simulink library "passive_control"  (Simulink 7.1)
values from neighbouring files (symbols this model uses):
  sysdsp = feedback(sysdp,Kc)    [calc_sysdsp.m]
  Ts = 1    [calc_sysdsp.m]
undefined symbols (not defined in the file or in its folder): A, B, b, C, D, gravload, Kv, Kx, M, ms, nc, np, q0, tau_passify
libraries: instrumentlib x8, passive_control x4, simulink x4, roblocks x2, dspsigops x2
(part 2 of 2)

== system passive_control/passify/ipesh_vel_est_2 ==
  u : Inport
  Embedded MATLAB Function : Stateflow chart
  Unit Delay : UnitDelay  X0=x0  SampleTime=-1
  y : Outport
  wires:
  Embedded MATLAB Function/1(y) -> y/1
  u/1 -> Embedded MATLAB Function/1(u)
  Unit Delay/1 -> Embedded MATLAB Function/2(x_k)
  Embedded MATLAB Function/2(x_k_p_1) -> Unit Delay/1

== system passive_control/passify/ipesh_vel_est_3 ==
  u : Inport
  Embedded MATLAB Function : Stateflow chart
  Unit Delay : UnitDelay  X0=x0  SampleTime=-1
  y : Outport
  wires:
  Embedded MATLAB Function/2(x_k_p_1) -> Unit Delay/1
  Unit Delay/1 -> Embedded MATLAB Function/2(x_k)
  u/1 -> Embedded MATLAB Function/1(u)
  Embedded MATLAB Function/1(y) -> y/1

== system passive_control/passify/ipesh_vel_est_4 ==
  u : Inport
  Embedded MATLAB Function : Stateflow chart
  Unit Delay : UnitDelay  X0=x0  SampleTime=-1
  y : Outport
  wires:
  Embedded MATLAB Function/1(y) -> y/1
  u/1 -> Embedded MATLAB Function/1(u)
  Unit Delay/1 -> Embedded MATLAB Function/2(x_k)
  Embedded MATLAB Function/2(x_k_p_1) -> Unit Delay/1

== system passive_control/passive_down_sampler/DT_Integrator ==
  In1 : Inport
  Sum2 : Sum  Inputs=|++  OutDataType=sfix(16)  OutScaling=2^0
  Unit Delay : UnitDelay  Orientation=left  SampleTime=-1
  Out1 : Outport
  wires:
  In1/1 -> Sum2/1
  Unit Delay/1 -> Sum2/2
  Sum2/1 -> Out1/1, Unit Delay/1  "sum_1"

== system passive_control/passive_down_sampler/DT_Integrator1 ==
  In1 : Inport
  Sum2 : Sum  Inputs=|++  OutDataType=sfix(16)  OutScaling=2^0
  Unit Delay : UnitDelay  Orientation=left  SampleTime=-1
  Out1 : Outport
  wires:
  Sum2/1 -> Unit Delay/1, Out1/1  "sum_1"
  Unit Delay/1 -> Sum2/2
  In1/1 -> Sum2/1

== system passive_control/trajectory_gen/ipesh_traj ==
  u : Inport
  Embedded MATLAB Function : Stateflow chart
  Unit Delay : UnitDelay  X0=x0  SampleTime=-1
  y : Outport
  wires:
  Embedded MATLAB Function/1(y) -> y/1
  u/1 -> Embedded MATLAB Function/1(u)
  Unit Delay/1 -> Embedded MATLAB Function/2(x_k)
  Embedded MATLAB Function/2(x_k_p_1) -> Unit Delay/1

== system passive_control/trajectory_gen/ipesh_traj1 ==
  u : Inport
  Embedded MATLAB Function : Stateflow chart
  Unit Delay : UnitDelay  X0=x0  SampleTime=-1
  y : Outport
  wires:
  Embedded MATLAB Function/2(x_k_p_1) -> Unit Delay/1
  Unit Delay/1 -> Embedded MATLAB Function/2(x_k)
  u/1 -> Embedded MATLAB Function/1(u)
  Embedded MATLAB Function/1(y) -> y/1

== system passive_control/trajectory_gen/ipesh_traj2 ==
  u : Inport
  Embedded MATLAB Function : Stateflow chart
  Unit Delay : UnitDelay  X0=x0  SampleTime=-1
  y : Outport
  wires:
  Embedded MATLAB Function/1(y) -> y/1
  u/1 -> Embedded MATLAB Function/1(u)
  Unit Delay/1 -> Embedded MATLAB Function/2(x_k)
  Embedded MATLAB Function/2(x_k_p_1) -> Unit Delay/1

== system passive_control/trajectory_gen/ipesh_traj3 ==
  u : Inport
  Embedded MATLAB Function : Stateflow chart
  Unit Delay : UnitDelay  X0=x0  SampleTime=-1
  y : Outport
  wires:
  Embedded MATLAB Function/2(x_k_p_1) -> Unit Delay/1
  Unit Delay/1 -> Embedded MATLAB Function/2(x_k)
  u/1 -> Embedded MATLAB Function/1(u)
  Embedded MATLAB Function/1(y) -> y/1

== system passive_control/Crustcrawler Robot/vel_est/ipesh_vel_est_1 ==
  u : Inport
  Embedded MATLAB Function : Stateflow chart
  Unit Delay : UnitDelay  Orientation=left  X0=x0  SampleTime=-1
  y : Outport
  wires:
  Embedded MATLAB Function/2(x_k_p_1) -> Unit Delay/1
  Unit Delay/1 -> Embedded MATLAB Function/2(x_k)
  u/1 -> Embedded MATLAB Function/1(u)
  Embedded MATLAB Function/1(y) -> y/1

== system passive_control/Crustcrawler Robot/vel_est/ipesh_vel_est_2 ==
  u : Inport
  Embedded MATLAB Function : Stateflow chart
  Unit Delay : UnitDelay  Orientation=left  X0=x0  SampleTime=-1
  y : Outport
  wires:
  Embedded MATLAB Function/1(y) -> y/1
  u/1 -> Embedded MATLAB Function/1(u)
  Unit Delay/1 -> Embedded MATLAB Function/2(x_k)
  Embedded MATLAB Function/2(x_k_p_1) -> Unit Delay/1

== system passive_control/Crustcrawler Robot/vel_est/ipesh_vel_est_3 ==
  u : Inport
  Embedded MATLAB Function : Stateflow chart
  Unit Delay : UnitDelay  Orientation=left  X0=x0  SampleTime=-1
  y : Outport
  wires:
  Embedded MATLAB Function/2(x_k_p_1) -> Unit Delay/1
  Unit Delay/1 -> Embedded MATLAB Function/2(x_k)
  u/1 -> Embedded MATLAB Function/1(u)
  Embedded MATLAB Function/1(y) -> y/1

== system passive_control/Crustcrawler Robot/vel_est/ipesh_vel_est_4 ==
  u : Inport
  Embedded MATLAB Function : Stateflow chart
  Unit Delay : UnitDelay  Orientation=left  X0=x0  SampleTime=-1
  y : Outport
  wires:
  Embedded MATLAB Function/1(y) -> y/1
  u/1 -> Embedded MATLAB Function/1(u)
  Unit Delay/1 -> Embedded MATLAB Function/2(x_k)
  Embedded MATLAB Function/2(x_k_p_1) -> Unit Delay/1

== system passive_control/Kp_Kv_CrustCrawler/trajectory_gen/ipesh_traj ==
  u : Inport
  Embedded MATLAB Function : Stateflow chart
  Unit Delay : UnitDelay  X0=x0  SampleTime=-1
  y : Outport
  wires:
  Embedded MATLAB Function/1(y) -> y/1
  u/1 -> Embedded MATLAB Function/1(u)
  Unit Delay/1 -> Embedded MATLAB Function/2(x_k)
  Embedded MATLAB Function/2(x_k_p_1) -> Unit Delay/1

== system passive_control/Kp_Kv_CrustCrawler/trajectory_gen/ipesh_traj1 ==
  u : Inport
  Embedded MATLAB Function : Stateflow chart
  Unit Delay : UnitDelay  X0=x0  SampleTime=-1
  y : Outport
  wires:
  Embedded MATLAB Function/2(x_k_p_1) -> Unit Delay/1
  Unit Delay/1 -> Embedded MATLAB Function/2(x_k)
  u/1 -> Embedded MATLAB Function/1(u)
  Embedded MATLAB Function/1(y) -> y/1

== system passive_control/Kp_Kv_CrustCrawler/trajectory_gen/ipesh_traj2 ==
  u : Inport
  Embedded MATLAB Function : Stateflow chart
  Unit Delay : UnitDelay  X0=x0  SampleTime=-1
  y : Outport
  wires:
  Embedded MATLAB Function/1(y) -> y/1
  u/1 -> Embedded MATLAB Function/1(u)
  Unit Delay/1 -> Embedded MATLAB Function/2(x_k)
  Embedded MATLAB Function/2(x_k_p_1) -> Unit Delay/1

== system passive_control/Kp_Kv_CrustCrawler/trajectory_gen/ipesh_traj3 ==
  u : Inport
  Embedded MATLAB Function : Stateflow chart
  Unit Delay : UnitDelay  X0=x0  SampleTime=-1
  y : Outport
  wires:
  Embedded MATLAB Function/2(x_k_p_1) -> Unit Delay/1
  Unit Delay/1 -> Embedded MATLAB Function/2(x_k)
  u/1 -> Embedded MATLAB Function/1(u)
  Embedded MATLAB Function/1(y) -> y/1

== system passive_control/Kp_Kv_CrustCrawler/vel_est/ipesh_vel_est_1 ==
  u : Inport
  Embedded MATLAB Function : Stateflow chart
  Unit Delay : UnitDelay  X0=x0  SampleTime=-1
  y : Outport
  wires:
  Embedded MATLAB Function/1(y) -> y/1
  u/1 -> Embedded MATLAB Function/1(u)
  Unit Delay/1 -> Embedded MATLAB Function/2(x_k)
  Embedded MATLAB Function/2(x_k_p_1) -> Unit Delay/1

== system passive_control/Kp_Kv_CrustCrawler/vel_est/ipesh_vel_est_2 ==
  u : Inport
  Embedded MATLAB Function : Stateflow chart
  Unit Delay : UnitDelay  X0=x0  SampleTime=-1
  y : Outport
  wires:
  Embedded MATLAB Function/2(x_k_p_1) -> Unit Delay/1
  Unit Delay/1 -> Embedded MATLAB Function/2(x_k)
  u/1 -> Embedded MATLAB Function/1(u)
  Embedded MATLAB Function/1(y) -> y/1

== system passive_control/Kp_Kv_CrustCrawler/vel_est/ipesh_vel_est_3 ==
  u : Inport
  Embedded MATLAB Function : Stateflow chart
  Unit Delay : UnitDelay  X0=x0  SampleTime=-1
  y : Outport
  wires:
  Embedded MATLAB Function/1(y) -> y/1
  u/1 -> Embedded MATLAB Function/1(u)
  Unit Delay/1 -> Embedded MATLAB Function/2(x_k)
  Embedded MATLAB Function/2(x_k_p_1) -> Unit Delay/1

== system passive_control/Kp_Kv_CrustCrawler/vel_est/ipesh_vel_est_4 ==
  u : Inport
  Embedded MATLAB Function : Stateflow chart
  Unit Delay : UnitDelay  X0=x0  SampleTime=-1
  y : Outport
  wires:
  Embedded MATLAB Function/2(x_k_p_1) -> Unit Delay/1
  Unit Delay/1 -> Embedded MATLAB Function/2(x_k)
  u/1 -> Embedded MATLAB Function/1(u)
  Embedded MATLAB Function/1(y) -> y/1

== matlab function passive_up_sampler/M_sample_hold ==
  data: u input double size=[N]; y output double size=[N]; M parameter double size=1; N parameter double size=1
function y = fcn(u, M, N)
persistent u_c;
   [m,n]=size(u);
   if m < n
       u = u';
       m = n;
       tra=true;
   else
       tra=false;
   end
   if isempty(u_c)    
       u_c = zeros(m,max(1,M-1));
   end
   y = u;
   for i = 1:(M-1)
       y = y + u_c(:,i);
   end
   for i = (M-1):-1:2
       u_c(:,i)=u_c(:,i-1);
   end
   u_c(:,1)=u;
   if tra
       y = y';
   end

== matlab function ipesh_abcd/Embedded MATLAB Function ==
  settings: updateMethod=DISCRETE  sampleTime=Ts
  data: u input single size=[1]; y output double size=[1]; x_k input single; x_k_p_1 output double; A parameter double; B parameter double; C parameter double; D parameter double
function [y,x_k_p_1] = fcn(u, x_k, A, B, C, D)
% This block supports the Embedded MATLAB subset.
% See the help menu for details. 
    x_k_p_1=A*x_k + B*u;
    y = C*x_k + D*u;

== matlab function Crustcrawler Robot/vel_est/ipesh_vel_est_1/Embedded MATLAB Function ==
  settings: updateMethod=DISCRETE  sampleTime=Ts
  data: u input single size=[1]; y output double size=[1]; x_k input single; x_k_p_1 output double; A parameter double; B parameter double; C parameter double; D parameter double
function [y,x_k_p_1] = fcn(u, x_k, A, B, C, D)
% This block supports the Embedded MATLAB subset.
% See the help menu for details. 
    x_k_p_1=A*x_k + B*u;
    y = C*x_k + D*u;

== matlab function Crustcrawler Robot/vel_est/ipesh_vel_est_2/Embedded MATLAB Function ==
  settings: updateMethod=DISCRETE  sampleTime=Ts
  data: u input single size=[1]; y output double size=[1]; x_k input single; x_k_p_1 output double; A parameter double; B parameter double; C parameter double; D parameter double
function [y,x_k_p_1] = fcn(u, x_k, A, B, C, D)
% This block supports the Embedded MATLAB subset.
% See the help menu for details. 
    x_k_p_1=A*x_k + B*u;
    y = C*x_k + D*u;

== matlab function Crustcrawler Robot/vel_est/ipesh_vel_est_3/Embedded MATLAB Function ==
  settings: updateMethod=DISCRETE  sampleTime=Ts
  data: u input single size=[1]; y output double size=[1]; x_k input single; x_k_p_1 output double; A parameter double; B parameter double; C parameter double; D parameter double
function [y,x_k_p_1] = fcn(u, x_k, A, B, C, D)
% This block supports the Embedded MATLAB subset.
% See the help menu for details. 
    x_k_p_1=A*x_k + B*u;
    y = C*x_k + D*u;

== matlab function Crustcrawler Robot/vel_est/ipesh_vel_est_4/Embedded MATLAB Function ==
  settings: updateMethod=DISCRETE  sampleTime=Ts
  data: u input single size=[1]; y output double size=[1]; x_k input single; x_k_p_1 output double; A parameter double; B parameter double; C parameter double; D parameter double
function [y,x_k_p_1] = fcn(u, x_k, A, B, C, D)
% This block supports the Embedded MATLAB subset.
% See the help menu for details. 
    x_k_p_1=A*x_k + B*u;
    y = C*x_k + D*u;

== matlab function time_stamp/time_stamp ==
  data: u input double; y output double
function y = fcn(u)
% This block supports the Embedded MATLAB subset.
% See the help menu for details.
y=zeros(1,6+length(u));
y(1:6)=feval('clock');
y(7:6+length(u)) = u;

== matlab function cc_wave_filter/ipesh_abcd/Embedded MATLAB Function ==
  settings: updateMethod=DISCRETE  sampleTime=Ts
  data: u input single size=[1]; y output double size=[1]; x_k input single; x_k_p_1 output double; A parameter double; B parameter double; C parameter double; D parameter double
function [y,x_k_p_1] = fcn(u, x_k, A, B, C, D)
% This block supports the Embedded MATLAB subset.
% See the help menu for details. 
    x_k_p_1=A*x_k + B*u;
    y = C*x_k + D*u;

== matlab function cc_wave_filter/ipesh_abcd1/Embedded MATLAB Function ==
  settings: updateMethod=DISCRETE  sampleTime=Ts
  data: u input single size=[1]; y output double size=[1]; x_k input single; x_k_p_1 output double; A parameter double; B parameter double; C parameter double; D parameter double
function [y,x_k_p_1] = fcn(u, x_k, A, B, C, D)
% This block supports the Embedded MATLAB subset.
% See the help menu for details. 
    x_k_p_1=A*x_k + B*u;
    y = C*x_k + D*u;

== matlab function Kp_Kv_CrustCrawler/trajectory_gen/ipesh_traj/Embedded MATLAB Function ==
  settings: updateMethod=DISCRETE  sampleTime=Ts
  data: u input single size=[1]; y output double size=[1]; x_k input single; x_k_p_1 output double; A parameter double; B parameter double; C parameter double; D parameter double
function [y,x_k_p_1] = fcn(u, x_k, A, B, C, D)
% This block supports the Embedded MATLAB subset.
% See the help menu for details. 
    x_k_p_1=A*x_k + B*u;
    y = C*x_k + D*u;

== matlab function Kp_Kv_CrustCrawler/trajectory_gen/ipesh_traj1/Embedded MATLAB Function ==
  settings: updateMethod=DISCRETE  sampleTime=Ts
  data: u input single size=[1]; y output double size=[1]; x_k input single; x_k_p_1 output double; A parameter double; B parameter double; C parameter double; D parameter double
function [y,x_k_p_1] = fcn(u, x_k, A, B, C, D)
% This block supports the Embedded MATLAB subset.
% See the help menu for details. 
    x_k_p_1=A*x_k + B*u;
    y = C*x_k + D*u;

== matlab function Kp_Kv_CrustCrawler/trajectory_gen/ipesh_traj2/Embedded MATLAB Function ==
  settings: updateMethod=DISCRETE  sampleTime=Ts
  data: u input single size=[1]; y output double size=[1]; x_k input single; x_k_p_1 output double; A parameter double; B parameter double; C parameter double; D parameter double
function [y,x_k_p_1] = fcn(u, x_k, A, B, C, D)
% This block supports the Embedded MATLAB subset.
% See the help menu for details. 
    x_k_p_1=A*x_k + B*u;
    y = C*x_k + D*u;

== matlab function cc_wave_filter/ipesh_abcd2/Embedded MATLAB Function ==
  settings: updateMethod=DISCRETE  sampleTime=Ts
  data: u input single size=[1]; y output double size=[1]; x_k input single; x_k_p_1 output double; A parameter double; B parameter double; C parameter double; D parameter double
function [y,x_k_p_1] = fcn(u, x_k, A, B, C, D)
% This block supports the Embedded MATLAB subset.
% See the help menu for details. 
    x_k_p_1=A*x_k + B*u;
    y = C*x_k + D*u;

== matlab function cc_wave_filter/ipesh_abcd3/Embedded MATLAB Function ==
  settings: updateMethod=DISCRETE  sampleTime=Ts
  data: u input single size=[1]; y output double size=[1]; x_k input single; x_k_p_1 output double; A parameter double; B parameter double; C parameter double; D parameter double
function [y,x_k_p_1] = fcn(u, x_k, A, B, C, D)
% This block supports the Embedded MATLAB subset.
% See the help menu for details. 
    x_k_p_1=A*x_k + B*u;
    y = C*x_k + D*u;

== matlab function Kp_Kv_CrustCrawler/trajectory_gen/ipesh_traj3/Embedded MATLAB Function ==
  settings: updateMethod=DISCRETE  sampleTime=Ts
  data: u input single size=[1]; y output double size=[1]; x_k input single; x_k_p_1 output double; A parameter double; B parameter double; C parameter double; D parameter double
function [y,x_k_p_1] = fcn(u, x_k, A, B, C, D)
% This block supports the Embedded MATLAB subset.
% See the help menu for details. 
    x_k_p_1=A*x_k + B*u;
    y = C*x_k + D*u;

== matlab function Kp_Kv_CrustCrawler/vel_est/ipesh_vel_est_1/Embedded MATLAB Function ==
  settings: updateMethod=DISCRETE  sampleTime=Ts
  data: u input single size=[1]; y output double size=[1]; x_k input single; x_k_p_1 output double; A parameter double; B parameter double; C parameter double; D parameter double
function [y,x_k_p_1] = fcn(u, x_k, A, B, C, D)
% This block supports the Embedded MATLAB subset.
% See the help menu for details. 
    x_k_p_1=A*x_k + B*u;
    y = C*x_k + D*u;

== matlab function Kp_Kv_CrustCrawler/vel_est/ipesh_vel_est_2/Embedded MATLAB Function ==
  settings: updateMethod=DISCRETE  sampleTime=Ts
  data: u input single size=[1]; y output double size=[1]; x_k input single; x_k_p_1 output double; A parameter double; B parameter double; C parameter double; D parameter double
function [y,x_k_p_1] = fcn(u, x_k, A, B, C, D)
% This block supports the Embedded MATLAB subset.
% See the help menu for details. 
    x_k_p_1=A*x_k + B*u;
    y = C*x_k + D*u;

== matlab function Kp_Kv_CrustCrawler/vel_est/ipesh_vel_est_3/Embedded MATLAB Function ==
  settings: updateMethod=DISCRETE  sampleTime=Ts
  data: u input single size=[1]; y output double size=[1]; x_k input single; x_k_p_1 output double; A parameter double; B parameter double; C parameter double; D parameter double
function [y,x_k_p_1] = fcn(u, x_k, A, B, C, D)
% This block supports the Embedded MATLAB subset.
% See the help menu for details. 
    x_k_p_1=A*x_k + B*u;
    y = C*x_k + D*u;

== matlab function Kp_Kv_CrustCrawler/vel_est/ipesh_vel_est_4/Embedded MATLAB Function ==
  settings: updateMethod=DISCRETE  sampleTime=Ts
  data: u input single size=[1]; y output double size=[1]; x_k input single; x_k_p_1 output double; A parameter double; B parameter double; C parameter double; D parameter double
function [y,x_k_p_1] = fcn(u, x_k, A, B, C, D)
% This block supports the Embedded MATLAB subset.
% See the help menu for details. 
    x_k_p_1=A*x_k + B*u;
    y = C*x_k + D*u;

== matlab function connect_to_pj/connect_to_pj ==
  data: w_o input double; w_o_r output double size=[4]; w_i input double; w_i_r output double size=[4]; connect parameter double
function [w_o_r,w_i_r] = fcn(w_o, w_i, connect)
% This block supports the Embedded MATLAB subset.
% See the help menu for details. 
if connect
    w_o_r = w_o;
    w_i_r = w_i;
else
    w_o_r = 0*w_o;
    w_i_r = 0*w_i;
end

== matlab function trajectory_gen/ipesh_traj/Embedded MATLAB Function ==
  settings: updateMethod=DISCRETE  sampleTime=Ts
  data: u input single size=[1]; y output double size=[1]; x_k input single; x_k_p_1 output double; A parameter double; B parameter double; C parameter double; D parameter double
function [y,x_k_p_1] = fcn(u, x_k, A, B, C, D)
% This block supports the Embedded MATLAB subset.
% See the help menu for details. 
    x_k_p_1=A*x_k + B*u;
    y = C*x_k + D*u;

== matlab function trajectory_gen/ipesh_traj1/Embedded MATLAB Function ==
  settings: updateMethod=DISCRETE  sampleTime=Ts
  data: u input single size=[1]; y output double size=[1]; x_k input single; x_k_p_1 output double; A parameter double; B parameter double; C parameter double; D parameter double
function [y,x_k_p_1] = fcn(u, x_k, A, B, C, D)
% This block supports the Embedded MATLAB subset.
% See the help menu for details. 
    x_k_p_1=A*x_k + B*u;
    y = C*x_k + D*u;

== matlab function trajectory_gen/ipesh_traj2/Embedded MATLAB Function ==
  settings: updateMethod=DISCRETE  sampleTime=Ts
  data: u input single size=[1]; y output double size=[1]; x_k input single; x_k_p_1 output double; A parameter double; B parameter double; C parameter double; D parameter double
function [y,x_k_p_1] = fcn(u, x_k, A, B, C, D)
% This block supports the Embedded MATLAB subset.
% See the help menu for details. 
    x_k_p_1=A*x_k + B*u;
    y = C*x_k + D*u;

== matlab function trajectory_gen/ipesh_traj3/Embedded MATLAB Function ==
  settings: updateMethod=DISCRETE  sampleTime=Ts
  data: u input single size=[1]; y output double size=[1]; x_k input single; x_k_p_1 output double; A parameter double; B parameter double; C parameter double; D parameter double
function [y,x_k_p_1] = fcn(u, x_k, A, B, C, D)
% This block supports the Embedded MATLAB subset.
% See the help menu for details. 
    x_k_p_1=A*x_k + B*u;
    y = C*x_k + D*u;

== matlab function passify/ipesh_vel_est_1/Embedded MATLAB Function ==
  settings: updateMethod=DISCRETE  sampleTime=Ts
  data: u input single size=[1]; y output double size=[1]; x_k input single; x_k_p_1 output double; A parameter double; B parameter double; C parameter double; D parameter double
function [y,x_k_p_1] = fcn(u, x_k, A, B, C, D)
% This block supports the Embedded MATLAB subset.
% See the help menu for details. 
    x_k_p_1=A*x_k + B*u;
    y = C*x_k + D*u;

== matlab function passify/ipesh_vel_est_2/Embedded MATLAB Function ==
  settings: updateMethod=DISCRETE  sampleTime=Ts
  data: u input single size=[1]; y output double size=[1]; x_k input single; x_k_p_1 output double; A parameter double; B parameter double; C parameter double; D parameter double
function [y,x_k_p_1] = fcn(u, x_k, A, B, C, D)
% This block supports the Embedded MATLAB subset.
% See the help menu for details. 
    x_k_p_1=A*x_k + B*u;
    y = C*x_k + D*u;

== matlab function passify/ipesh_vel_est_3/Embedded MATLAB Function ==
  settings: updateMethod=DISCRETE  sampleTime=Ts
  data: u input single size=[1]; y output double size=[1]; x_k input single; x_k_p_1 output double; A parameter double; B parameter double; C parameter double; D parameter double
function [y,x_k_p_1] = fcn(u, x_k, A, B, C, D)
% This block supports the Embedded MATLAB subset.
% See the help menu for details. 
    x_k_p_1=A*x_k + B*u;
    y = C*x_k + D*u;

== matlab function passify/ipesh_vel_est_4/Embedded MATLAB Function ==
  settings: updateMethod=DISCRETE  sampleTime=Ts
  data: u input single size=[1]; y output double size=[1]; x_k input single; x_k_p_1 output double; A parameter double; B parameter double; C parameter double; D parameter double
function [y,x_k_p_1] = fcn(u, x_k, A, B, C, D)
% This block supports the Embedded MATLAB subset.
% See the help menu for details. 
    x_k_p_1=A*x_k + B*u;
    y = C*x_k + D*u;

== matlab function lag_compensator/lag_compen/Embedded MATLAB Function ==
  settings: updateMethod=DISCRETE  sampleTime=Ts
  data: u input single size=[1]; y output double size=[1]; x_k input single; x_k_p_1 output double; A parameter double; B parameter double; C parameter double; D parameter double
function [y,x_k_p_1] = fcn(u, x_k, A, B, C, D)
% This block supports the Embedded MATLAB subset.
% See the help menu for details. 
    x_k_p_1=A*x_k + B*u;
    y = C*x_k + D*u;

== matlab function lag_compensator/lag_compen1/Embedded MATLAB Function ==
  settings: updateMethod=DISCRETE  sampleTime=Ts
  data: u input single size=[1]; y output double size=[1]; x_k input single; x_k_p_1 output double; A parameter double; B parameter double; C parameter double; D parameter double
function [y,x_k_p_1] = fcn(u, x_k, A, B, C, D)
% This block supports the Embedded MATLAB subset.
% See the help menu for details. 
    x_k_p_1=A*x_k + B*u;
    y = C*x_k + D*u;

== matlab function lag_compensator/lag_compen2/Embedded MATLAB Function ==
  settings: updateMethod=DISCRETE  sampleTime=Ts
  data: u input single size=[1]; y output double size=[1]; x_k input single; x_k_p_1 output double; A parameter double; B parameter double; C parameter double; D parameter double
function [y,x_k_p_1] = fcn(u, x_k, A, B, C, D)
% This block supports the Embedded MATLAB subset.
% See the help menu for details. 
    x_k_p_1=A*x_k + B*u;
    y = C*x_k + D*u;

== matlab function lag_compensator/lag_compen3/Embedded MATLAB Function ==
  settings: updateMethod=DISCRETE  sampleTime=Ts
  data: u input single size=[1]; y output double size=[1]; x_k input single; x_k_p_1 output double; A parameter double; B parameter double; C parameter double; D parameter double
function [y,x_k_p_1] = fcn(u, x_k, A, B, C, D)
% This block supports the Embedded MATLAB subset.
% See the help menu for details. 
    x_k_p_1=A*x_k + B*u;
    y = C*x_k + D*u;

== matlab function passive_down_sampler/pass_through ==
  data: u input double; y output double; M parameter double
function y = fcn(u, M)
% This block supports the Embedded MATLAB subset.
% See the help menu for details. 
if M == 1
    y = u;
else
    y = 0*u;
end
